simulink model "Realimentacion_Estados"  (R2021a)
settings: Solver=VariableStepAuto  StartTime=0.0  StopTime=10.0  RelTol=1e-3
values from neighbouring files (symbols this model uses):
  K = Ka(1:3)    [TP1.m]
  kI = -Ka(end)    [TP1.m]
settings Model: Creator=Euge Etcheverry  LastModifiedBy=Euge Etcheverry

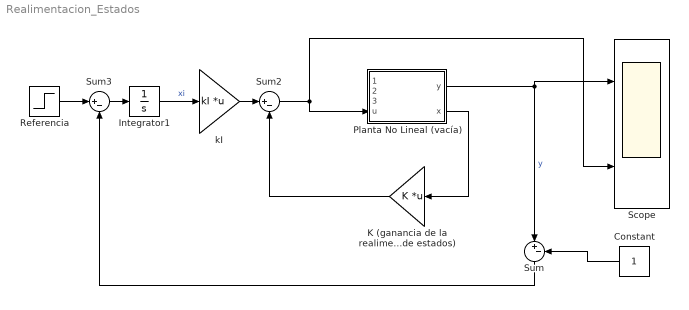
== system Realimentacion_Estados ==
  Constant : Constant
  Integrator1 : Integrator
  K (ganancia de la realimentacion de estados) : Gain  Gain=K  Multiplication=Matrix(K*u)
  Planta No Lineal (vacía) : Subsystem
  Referencia : Step  After=0.5  SampleTime=0
  Scope : Scope  NumInputPorts=2
  Sum : Sum  Inputs=|+-
  Sum2 : Sum  Inputs=|+-
  Sum3 : Sum  Inputs=|+-
  kI : Gain  Gain=kI  Multiplication=Matrix(K*u)
  wires:
  Sum3/1 -> Integrator1/1
  Referencia/1 -> Sum3/1
  Planta No Lineal (vacía)/1(y) -> Sum/1, Scope/1  "y"
  Constant/1 -> Sum/2
  kI/1 -> Sum2/1
  Integrator1/1 -> kI/1  "xi"
  Sum/1 -> Sum3/2
  Sum2/1 -> Scope/2, Planta No Lineal (vacía)/4(u)
  Planta No Lineal (vacía)/2(x) -> K (ganancia de la realimentacion de estados)/1
  K (ganancia de la realimentacion de estados)/1 -> Sum2/2

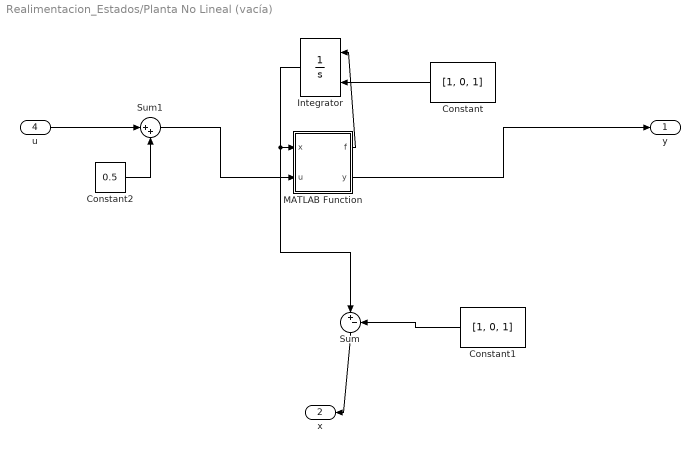
== system Realimentacion_Estados/Planta No Lineal (vacía) ==
  u : Inport  Port=4
  Constant : Constant  Value=[1, 0, 1]
  Constant1 : Constant  Value=[1, 0, 1]
  Constant2 : Constant  Value=0.5
  Integrator : Integrator  InitialConditionSource=external
  MATLAB Function : MATLAB Function  TreatAsAtomicUnit=on
  Sum : Sum  Inputs=|+-
  Sum1 : Sum  Inputs=|++
  y : Outport
  x : Outport  Port=2
  wires:
  MATLAB Function/1(f) -> Integrator/1
  Integrator/1 -> Sum/1, MATLAB Function/1(x)
  MATLAB Function/2(y) -> y/1
  Constant/1 -> Integrator/2
  Constant1/1 -> Sum/2
  Sum/1 -> x/1
  u/1 -> Sum1/1
  Sum1/1 -> MATLAB Function/2(u)
  Constant2/1 -> Sum1/2

== matlab function Realimentacion_Estados/Planta No Lineal (vacía)/MATLAB Function ==
  data: x input; f output; y output; u input
function [f,y] = fcn(x, u)

g = 10;
m = 0.1;
L = 1e-2;
R = 4;

f1=x(2);
f2=g-x(3)/(m*x(1));
f3=u/L-x(3)*R/L;

f=[f1;f2;f3];

y=x(1);
